simulink model "ControledLine11"  (R2015b)
settings: configuration reference "ControlConfig" (kept outside this file)
values from neighbouring files (symbols this model uses):
  Ts = 0.02    [ControlInit.m]
undefined symbols (not defined in the file or in its folder): DiscIntNeverNeededParam
libraries: powerlib x10, simulink x4, powerlib_meascontrol x1
settings Model: Creator=Emilio  LastModifiedBy=Emilio
settings ConfigSetRef: SourceLocation=Base Workspace

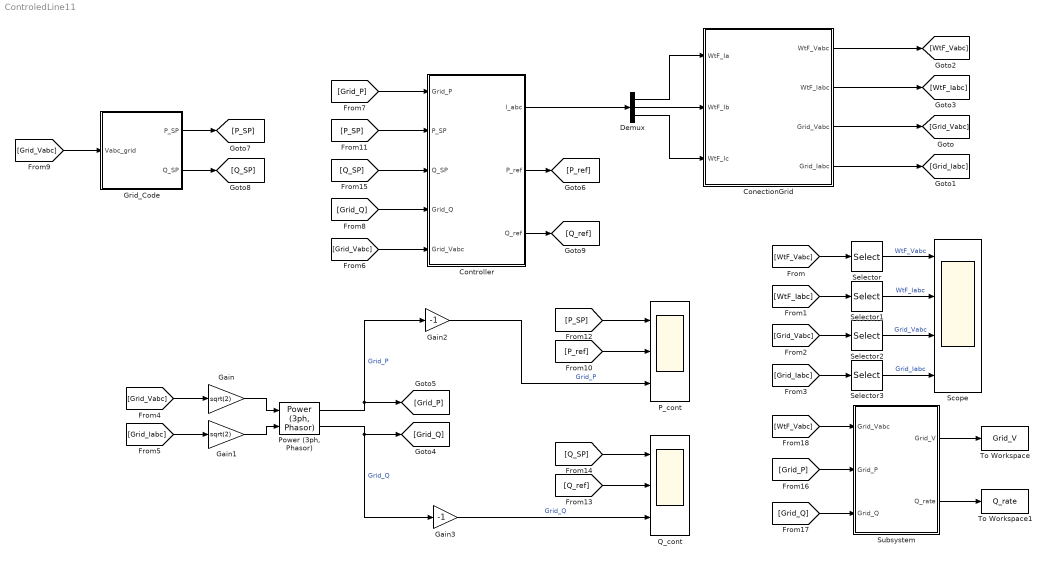
== system ControledLine11 ==
  ConectionGrid : Subsystem
  Controller : Subsystem
  Demux : Demux  Outputs=3
  Gain : Gain  Gain=sqrt(2)
  Gain1 : Gain  Gain=sqrt(2)
  Gain2 : Gain  Gain=-1
  Gain3 : Gain  Gain=-1
  Grid_Code : Subsystem
  P_cont : Scope  NumInputPorts=3
  "Power (3ph, Phasor)" : powerlib_meascontrol/Measurements/Power (3ph, Phasor)
  Q_cont : Scope  NumInputPorts=3
  Scope : Scope  NumInputPorts=4
  Selector{,1..3} (4 alike) : Selector  InputPortWidth=3  IndexOptions=Index vector (dialog)  Indices=[1]  OutputSizes=1
  Subsystem : Subsystem
  To Workspace : ToWorkspace  VariableName=Grid_V  SampleTime=Ts
  To Workspace1 : ToWorkspace  VariableName=Q_rate  SaveFormat=Timeseries  SampleTime=-1
  wires:
  ConectionGrid/1(WtF_Vabc) -> [WtF_Vabc]
  ConectionGrid/2(WtF_Iabc) -> [WtF_Iabc]
  ConectionGrid/3(Grid_Vabc) -> [Grid_Vabc]
  ConectionGrid/4(Grid_Iabc) -> [Grid_Iabc]
  [WtF_Vabc] -> Selector/1
  [WtF_Iabc] -> Selector1/1
  [Grid_Vabc] -> Selector2/1
  [Grid_Iabc] -> Selector3/1
  Selector/1 -> Scope/1  "WtF_Vabc"
  Selector1/1 -> Scope/2  "WtF_Iabc"
  Selector2/1 -> Scope/3  "Grid_Vabc"
  Selector3/1 -> Scope/4  "Grid_Iabc"
  [Grid_Vabc] -> Gain/1
  [Grid_Iabc] -> Gain1/1
  Gain/1 -> "Power (3ph, Phasor)"/1
  Gain1/1 -> "Power (3ph, Phasor)"/2
  "Power (3ph, Phasor)"/1 -> [Grid_P], Gain2/1  "Grid_P"
  "Power (3ph, Phasor)"/2 -> Gain3/1, [Grid_Q]  "Grid_Q"
  [Grid_Q] -> Controller/4(Grid_Q)
  [Grid_Vabc] -> Controller/5(Grid_Vabc)
  [Grid_P] -> Controller/1(Grid_P)
  Controller/1(I_abc) -> Demux/1
  Demux/1 -> ConectionGrid/1(WtF_Ia)
  Demux/2 -> ConectionGrid/2(WtF_Ib)
  Demux/3 -> ConectionGrid/3(WtF_Ic)
  [Grid_Vabc] -> Grid_Code/1(Vabc_grid)
  Gain2/1 -> P_cont/3  "Grid_P"
  Gain3/1 -> Q_cont/3  "Grid_Q"
  Controller/2(P_ref) -> [P_ref]
  [P_ref] -> P_cont/2
  Grid_Code/1(P_SP) -> [P_SP]
  [P_SP] -> Controller/2(P_SP)
  [P_SP] -> P_cont/1
  Grid_Code/2(Q_SP) -> [Q_SP]
  [Q_ref] -> Q_cont/2
  [Q_SP] -> Q_cont/1
  Controller/3(Q_ref) -> [Q_ref]
  [Q_SP] -> Controller/3(Q_SP)
  [Grid_P] -> Subsystem/2(Grid_P)
  [Grid_Q] -> Subsystem/3(Grid_Q)
  [WtF_Vabc] -> Subsystem/1(Grid_Vabc)
  Subsystem/2(Q_rate) -> To Workspace1/1
  Subsystem/1(Grid_V) -> To Workspace/1

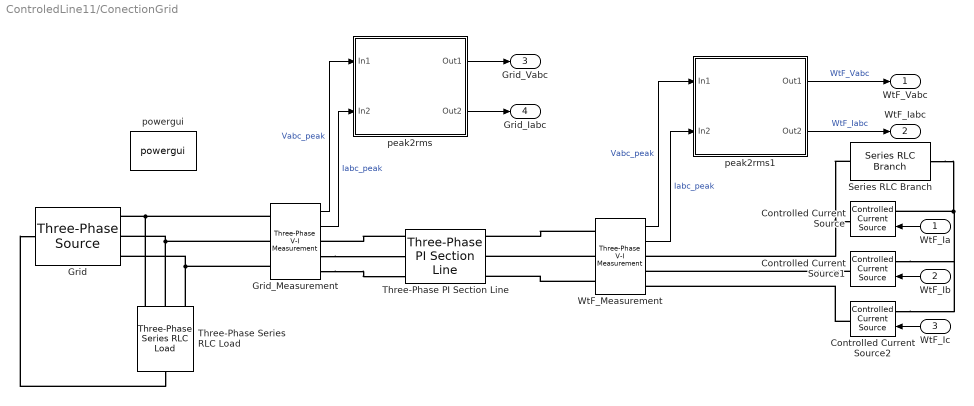
== system ControledLine11/ConectionGrid ==
  WtF_Ia : Inport
  WtF_Ib : Inport  Port=2
  WtF_Ic : Inport  Port=3
  Controlled Current Source : powerlib/Electrical Sources/Controlled Current Source  Initialize=on  Source_Type=AC  Amplitude=0  Phase=0  Frequency=50  Measurements=None
  Controlled Current Source1 : powerlib/Electrical Sources/Controlled Current Source  Initialize=on  Source_Type=AC  Amplitude=0  Phase=0  Frequency=50  Measurements=None
  Controlled Current Source2 : powerlib/Electrical Sources/Controlled Current Source  Initialize=on  Source_Type=AC  Amplitude=0  Phase=0  Frequency=50  Measurements=None
  Grid : powerlib/Electrical Sources/Three-Phase Source  InternalConnection=Yn  VoltagePhases=off  Voltage=400e3  PhaseAngle=0  Voltage_phases=[25e3 25e3 25e3]/sqrt(3)  PhaseAngles_phases=[0 -120 +120]  Frequency=50  NonIdealSource=on  SpecifyImpedance=on  Resistance=0.8929  Inductance=16.58e-3  ShortCircuitLevel=100e6  BaseVoltage=25e3  XRratio=7  BusType=swing  Pref=10e3  Qref=0  Prefabc=[10e3, 10e3, 10e3]  Qrefabc=[0, 0, 0]  Qmin=-inf  Qmax=inf
  Grid_Measurement : powerlib/Measurements/Three-Phase V-I Measurement  VoltageMeasurement=phase-to-ground  SetLabelV=off  LabelV=Vabc  Vpu=off  VpuLL=off  CurrentMeasurement=yes  SetLabelI=off  LabelI=Iabc  Ipu=off  Pbase=100e6  Vbase=500e3  OutputType=Complex  PhasorSimulation=on  PSBequivalent=0
  Series RLC Branch : powerlib/Elements/Series RLC Branch  LConnTagsString=__new0  RConnTagsString=__new0  BranchType=R  Resistance=10e10  Inductance=1e-3  SetiL0=off  InitialCurrent=0  Capacitance=1e-6  Setx0=off  InitialVoltage=0  Measurements=None
  Three-Phase PI Section Line : powerlib/Elements/Three-Phase PI Section Line  LConnTagsString=a|b|c  RConnTagsString=A|B|C  Frequency=60  Resistances=[ 0.01273 0.3864]  Inductances="[ 0.9337e-3  4.1264e-3]"  Capacitances=[12.74e-9 7.751e-9]  Length=100
  Three-Phase Series RLC Load : powerlib/Elements/Three-Phase Series RLC Load  LConnTagsString=A|B|C  RConnTagsString=N  Configuration=Y (neutral)  NominalVoltage=1000  Vabc=[1e3 1e3 1e3]  Vabcp=[1e3 1e3 1e3]  NominalFrequency=60  UnbalancedPower=off  ActivePower=10  InductivePower=0  CapacitivePower=0  Pabc=[10e3 9e3 11e3]  QLabc=[100 90 110]  QCabc=[100 90 110]  Pabcp=[10e3 9e3 11e3]  QLabcp=[100 90 110]  QCabcp=[100 90 110]  Measurements=None  LoadType=constant Z
  WtF_Measurement : powerlib/Measurements/Three-Phase V-I Measurement  VoltageMeasurement=phase-to-ground  SetLabelV=off  LabelV=Vabc  Vpu=off  VpuLL=off  CurrentMeasurement=yes  SetLabelI=off  LabelI=Iabc  Ipu=off  Pbase=100e6  Vbase=500e3  OutputType=Complex  PhasorSimulation=on  PSBequivalent=0
  peak2rms : Subsystem
  peak2rms1 : Subsystem
  powergui : powerlib/powergui  Priority=1  SimulationMode=Phasor  SolverType=Tustin/Backward Euler (TBE)  SampleTime=50e-6  frequency=50  SPID=off  DisableSnubberDevices=off  DisableRonSwitches=off  DisableVfSwitches=off  SwTol=0  DisplayEquations=off  Interpol=off  ExternalGateDelay=off  methode=off  Ts=10  FunctionMessages=off  echomessages=off  HookPort=off  EnableUseOfTLC=off  x0status=blocks  frequencyindice=50  Pbase=100e6  ErrMax=1e-4  Iterations=50  UnitsV=kV  UnitsW=MW  buscounter=0  RestoreLinks=warning  ResistiveCurrentMeasurement=off  Frange=[0:2:500]  Ylog=off  Xlog=on  ShowGrid=off  save=off  variable=ZData  structure=0  ZoomFFT=off  StartTime=0.0  cycles=1  DisplayStyle=1  fundamental=60  FreqAxis=off  MaxFrequency=1000  frequencyindicesteady=1  RmsSteady=1  display=off
  WtF_Vabc : Outport
  WtF_Iabc : Outport  Port=2
  Grid_Vabc : Outport  Port=3
  Grid_Iabc : Outport  Port=4
  wires:
  peak2rms/1(Out1) -> Grid_Vabc/1
  peak2rms/2(Out2) -> Grid_Iabc/1
  Grid_Measurement/2 -> peak2rms/2(In2)  "Iabc_peak"
  Grid_Measurement/1 -> peak2rms/1(In1)  "Vabc_peak"
  WtF_Measurement/2 -> peak2rms1/2(In2)  "Iabc_peak"
  peak2rms1/1(Out1) -> WtF_Vabc/1  "WtF_Vabc"
  peak2rms1/2(Out2) -> WtF_Iabc/1  "WtF_Iabc"
  WtF_Measurement/1 -> peak2rms1/1(In1)  "Vabc_peak"
  WtF_Ic/1 -> Controlled Current Source2/1
  WtF_Ib/1 -> Controlled Current Source1/1
  WtF_Ia/1 -> Controlled Current Source/1
  connections:
  Three-Phase Series RLC Load/LConn2 -- Grid/RConn2 -- Grid_Measurement/LConn2
  Grid_Measurement/RConn2 -- Three-Phase PI Section Line/LConn2
  Grid_Measurement/RConn3 -- Three-Phase PI Section Line/LConn3
  Series RLC Branch/LConn1 -- WtF_Measurement/RConn1 -- Controlled Current Source/RConn1
  WtF_Measurement/LConn2 -- Three-Phase PI Section Line/RConn2
  Controlled Current Source2/LConn1 -- Controlled Current Source1/LConn1 -- Series RLC Branch/RConn1 -- Controlled Current Source/LConn1
  WtF_Measurement/LConn3 -- Three-Phase PI Section Line/RConn3
  WtF_Measurement/LConn1 -- Three-Phase PI Section Line/RConn1
  Three-Phase Series RLC Load/LConn3 -- Grid/RConn3 -- Grid_Measurement/LConn3
  Three-Phase PI Section Line/LConn1 -- Grid_Measurement/RConn1
  Three-Phase Series RLC Load/LConn1 -- Grid/RConn1 -- Grid_Measurement/LConn1
  Controlled Current Source2/RConn1 -- WtF_Measurement/RConn3
  Controlled Current Source1/RConn1 -- WtF_Measurement/RConn2
  Three-Phase Series RLC Load/RConn1 -- Grid/LConn1

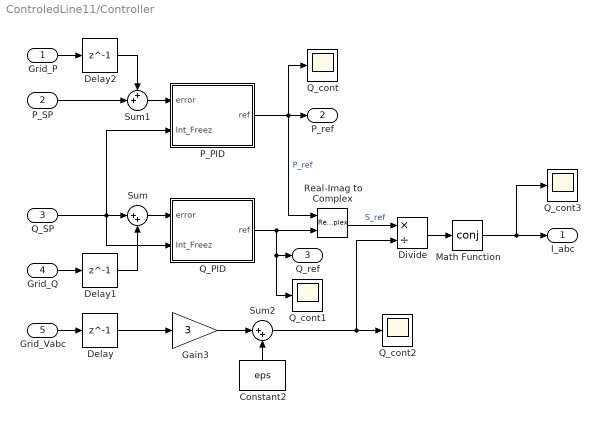
== system ControledLine11/Controller ==
  Grid_P : Inport
  P_SP : Inport  Port=2
  Q_SP : Inport  Port=3
  Grid_Q : Inport  Port=4
  Grid_Vabc : Inport  Port=5
  Constant2 : Constant  Value=eps
  Delay : Delay  DelayLength=1  InitialCondition=0
  Delay1 : Delay  DelayLength=1  InitialCondition=0
  Delay2 : Delay  DelayLength=1  InitialCondition=0
  Divide : Product  Inputs=*/
  Gain3 : Gain  Gain=3
  Math Function : Math  Operator=conj  SaturateOnIntegerOverflow=on
  P_PID : Subsystem
  Q_PID : Subsystem
  Q_cont{,1..3} (4 alike) : Scope
  Real-Imag to Complex : RealImagToComplex
  Sum : Sum  Inputs=|++
  Sum1 : Sum  Inputs=++|
  Sum2 : Sum  Inputs=|++
  I_abc : Outport
  P_ref : Outport  Port=2
  Q_ref : Outport  Port=3
  wires:
  Real-Imag to Complex/1 -> Divide/1  "S_ref"
  Grid_Q/1 -> Delay1/1
  Delay/1 -> Gain3/1
  Grid_Vabc/1 -> Delay/1
  Delay1/1 -> Sum/2
  P_PID/1(ref) -> Q_cont/1, P_ref/1, Real-Imag to Complex/1  "P_ref"
  Sum1/1 -> P_PID/1(error)
  P_SP/1 -> Sum1/2
  Grid_P/1 -> Delay2/1
  Delay2/1 -> Sum1/1
  Gain3/1 -> Sum2/1
  Constant2/1 -> Sum2/2
  Sum2/1 -> Q_cont2/1, Divide/2
  Divide/1 -> Math Function/1
  Q_PID/1(ref) -> Real-Imag to Complex/2, Q_cont1/1, Q_ref/1
  Q_SP/1 -> Q_PID/2(Int_Freez), P_PID/2(Int_Freez), Sum/1
  Math Function/1 -> I_abc/1, Q_cont3/1
  Sum/1 -> Q_PID/1(error)

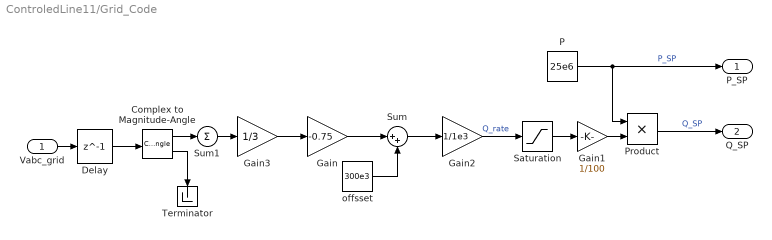
== system ControledLine11/Grid_Code ==
  Vabc_grid : Inport
  Complex to Magnitude-Angle : ComplexToMagnitudeAngle
  Delay : Delay  DelayLength=1
  Gain : Gain  Gain=-0.75
  Gain1 : Gain  Gain=1/100
  Gain2 : Gain  Gain=1/1e3
  Gain3 : Gain  Gain=1/3
  P : Constant  Value=25e6
  Product : Product
  Saturation : Saturate  UpperLimit=15  LowerLimit=-15
  Sum : Sum  Inputs=|++
  Sum1 : Sum  Inputs=+
  Terminator : Terminator
  offsset : Constant  Value=300e3
  P_SP : Outport
  Q_SP : Outport  Port=2
  wires:
  Product/1 -> Q_SP/1  "Q_SP"
  P/1 -> Product/1, P_SP/1  "P_SP"
  Gain/1 -> Sum/1
  offsset/1 -> Sum/2
  Sum/1 -> Gain2/1
  Vabc_grid/1 -> Delay/1
  Complex to Magnitude-Angle/1 -> Sum1/1
  Complex to Magnitude-Angle/2 -> Terminator/1
  Gain1/1 -> Product/2
  Delay/1 -> Complex to Magnitude-Angle/1
  Saturation/1 -> Gain1/1
  Gain2/1 -> Saturation/1  "Q_rate"
  Sum1/1 -> Gain3/1
  Gain3/1 -> Gain/1

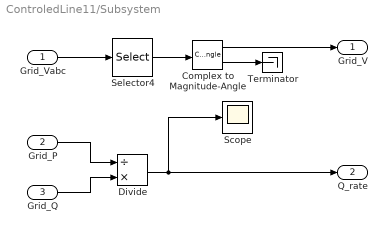
== system ControledLine11/Subsystem ==
  Grid_Vabc : Inport
  Grid_P : Inport  Port=2
  Grid_Q : Inport  Port=3
  Complex to Magnitude-Angle : ComplexToMagnitudeAngle
  Divide : Product  Inputs=/*
  Scope : Scope
  Selector4 : Selector  InputPortWidth=3  IndexOptions=Index vector (dialog)  Indices=[1]  OutputSizes=1
  Terminator : Terminator
  Grid_V : Outport
  Q_rate : Outport  Port=2
  wires:
  Divide/1 -> Q_rate/1, Scope/1
  Grid_P/1 -> Divide/1
  Selector4/1 -> Complex to Magnitude-Angle/1
  Grid_Vabc/1 -> Selector4/1
  Grid_Q/1 -> Divide/2
  Complex to Magnitude-Angle/2 -> Terminator/1
  Complex to Magnitude-Angle/1 -> Grid_V/1

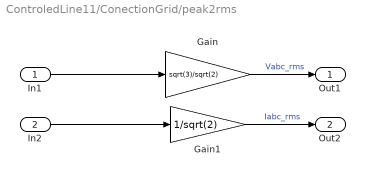
== system ControledLine11/ConectionGrid/peak2rms ==
  In1 : Inport
  In2 : Inport  Port=2
  Gain : Gain  Gain=sqrt(3)/sqrt(2)
  Gain1 : Gain  Gain=1/sqrt(2)
  Out1 : Outport
  Out2 : Outport  Port=2
  wires:
  Gain/1 -> Out1/1  "Vabc_rms"
  In1/1 -> Gain/1
  Gain1/1 -> Out2/1  "Iabc_rms"
  In2/1 -> Gain1/1

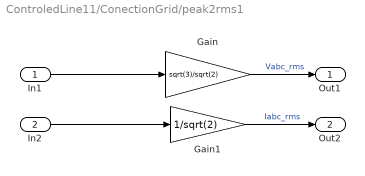
== system ControledLine11/ConectionGrid/peak2rms1 ==
  In1 : Inport
  In2 : Inport  Port=2
  Gain : Gain  Gain=sqrt(3)/sqrt(2)
  Gain1 : Gain  Gain=1/sqrt(2)
  Out1 : Outport
  Out2 : Outport  Port=2
  wires:
  In2/1 -> Gain1/1
  Gain1/1 -> Out2/1  "Iabc_rms"
  In1/1 -> Gain/1
  Gain/1 -> Out1/1  "Vabc_rms"

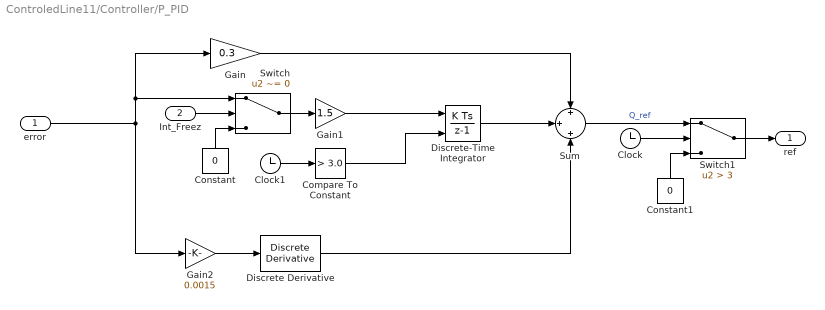
== system ControledLine11/Controller/P_PID ==
  error : Inport
  Int_Freez : Inport  Port=2
  Clock : Clock
  Clock1 : Clock
  Compare To Constant : simulink/Logic and Bit Operations/Compare To Constant  relop=>  const=3.0  OutDataTypeStr=boolean
  Constant : Constant  Value=0
  Constant1 : Constant  Value=0
  Discrete Derivative : simulink/Discrete/Discrete Derivative  gainval=1.0  ICPrevScaledInput=0.0  InputProcessing=Inherited  OutMin=[]  OutMax=[]  OutDataType=fixdt(1, 16)  OutScaling=2^-10  DoSatur=off
  Discrete-Time Integrator : DiscreteIntegrator  ExternalReset=rising  InitialConditionSetting=State (most efficient)  SampleTime=Ts  ICPrevOutput=DiscIntNeverNeededParam  ICPrevScaledInput=DiscIntNeverNeededParam
  Gain : Gain  Gain=0.3
  Gain1 : Gain  Gain=1.5
  Gain2 : Gain  Gain=0.0015
  Sum : Sum  Inputs=+|+|+
  Switch : Switch  Criteria=u2 ~= 0  Threshold=3
  Switch1 : Switch  Criteria=u2 > Threshold  Threshold=3
  ref : Outport
  wires:
  error/1 -> Gain2/1, Switch/1, Gain/1
  Switch/1 -> Gain1/1
  Constant/1 -> Switch/3
  Discrete Derivative/1 -> Sum/3
  Gain2/1 -> Discrete Derivative/1
  Gain1/1 -> Discrete-Time Integrator/1
  Gain/1 -> Sum/1
  Switch1/1 -> ref/1
  Constant1/1 -> Switch1/3
  Sum/1 -> Switch1/1  "Q_ref"
  Clock/1 -> Switch1/2
  Discrete-Time Integrator/1 -> Sum/2
  Clock1/1 -> Compare To Constant/1
  Compare To Constant/1 -> Discrete-Time Integrator/2
  Int_Freez/1 -> Switch/2

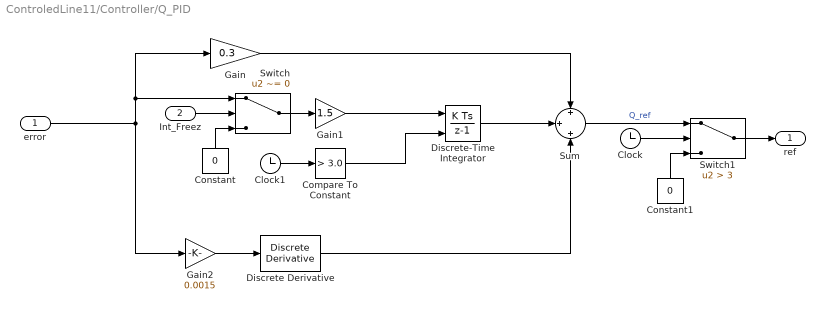
== system ControledLine11/Controller/Q_PID ==
  error : Inport
  Int_Freez : Inport  Port=2
  Clock : Clock
  Clock1 : Clock
  Compare To Constant : simulink/Logic and Bit Operations/Compare To Constant  relop=>  const=3.0  OutDataTypeStr=boolean
  Constant : Constant  Value=0
  Constant1 : Constant  Value=0
  Discrete Derivative : simulink/Discrete/Discrete Derivative  gainval=1.0  ICPrevScaledInput=0.0  InputProcessing=Inherited  OutMin=[]  OutMax=[]  OutDataType=fixdt(1, 16)  OutScaling=2^-10  DoSatur=off
  Discrete-Time Integrator : DiscreteIntegrator  ExternalReset=rising  InitialConditionSetting=State (most efficient)  SampleTime=Ts  ICPrevOutput=DiscIntNeverNeededParam  ICPrevScaledInput=DiscIntNeverNeededParam
  Gain : Gain  Gain=0.3
  Gain1 : Gain  Gain=1.5
  Gain2 : Gain  Gain=0.0015
  Sum : Sum  Inputs=+|+|+
  Switch : Switch  Criteria=u2 ~= 0  Threshold=3
  Switch1 : Switch  Criteria=u2 > Threshold  Threshold=3
  ref : Outport
  wires:
  Int_Freez/1 -> Switch/2
  Compare To Constant/1 -> Discrete-Time Integrator/2
  Clock1/1 -> Compare To Constant/1
  Discrete-Time Integrator/1 -> Sum/2
  Clock/1 -> Switch1/2
  Sum/1 -> Switch1/1  "Q_ref"
  Constant1/1 -> Switch1/3
  Switch1/1 -> ref/1
  Gain/1 -> Sum/1
  Gain1/1 -> Discrete-Time Integrator/1
  Gain2/1 -> Discrete Derivative/1
  Discrete Derivative/1 -> Sum/3
  Constant/1 -> Switch/3
  Switch/1 -> Gain1/1
  error/1 -> Gain/1, Switch/1, Gain2/1
